simulink model "Absolute_Time_Temporal_Logic"  (R2018b)
settings: Solver=FixedStepDiscrete  StartTime=0.0  StopTime=40.0  FixedStep=1  RelTol=1e-3
undefined symbols (not defined in the file or in its folder): sigbuilder_block
settings Model: Creator=marwan  LastModifiedBy=marwan

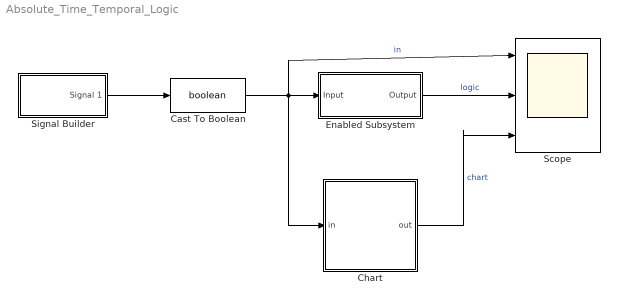
== system Absolute_Time_Temporal_Logic ==
  Cast To Boolean : DataTypeConversion  OutDataTypeStr=boolean
  Chart : Stateflow chart  TreatAsAtomicUnit=on
  Enabled Subsystem : Subsystem  TreatAsAtomicUnit=on
  Scope : Scope  NumInputPorts=3
  Signal Builder : Subsystem  Tag=STV Subsys  LoadFcn=sigbuilder_block('load');  StartFcn=sigbuilder_block('start');  StopFcn=sigbuilder_block('stop');  ClipboardFcn=sigbuilder_block('clipboard');  mask(Sigbuilder block){tuvar=[0:10]}
      mask help: Simulink:masks:SigbuilderBlock_MD
      mask init:
      | if ~strcmp(get_param(bdroot(gcbh),'SimulationStatus'),'stopped') tuvar = sigbuilder_block('maskInit'); end
      settings: CopyFcn=sigbuilder_block('copy');  DeleteFcn=sigbuilder_block('delete');  ModelCloseFcn=sigbuilder_block('modelClose');  PreSaveFcn=sigbuilder_block('preSave');  PauseFcn=sigbuilder_block('pause');  ContinueFcn=sigbuilder_block('continue');  NameChangeFcn=sigbuilder_block('namechange');  OpenFcn=sigbuilder_block('open',[369 79.5 565.5 358.5 ]);  CloseFcn=sigbuilder_block('close');
      mask Display: plot(0, 0, 100, 100,[2, 2, 32, 32, 2], [68, 8, 8, 68, 68],[32, 2], [38, 38], [32, 19, 2],[53, 60, 44], [32, 17, 17, 2],[16, 16, 31, 31]);txt = getActiveGroup(gcbh);text(2, 100, txt,'verticalAlignment', 'top');
  wires:
  Signal Builder/1(Signal 1) -> Cast To Boolean/1
  Cast To Boolean/1 -> Chart/1(in), Scope/1, Enabled Subsystem/1(Input)  "in"
  Enabled Subsystem/1(Output) -> Scope/2  "logic"
  Chart/1(out) -> Scope/3  "chart"

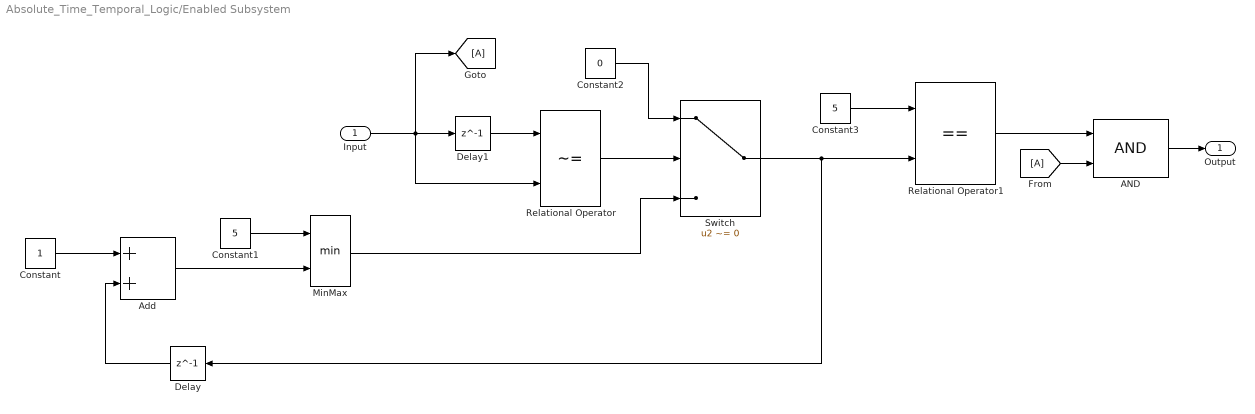
== system Absolute_Time_Temporal_Logic/Enabled Subsystem ==
  Input : Inport
  AND : Logic  IconShape=distinctive  AllPortsSameDT=off  OutDataTypeStr=boolean
  Add : Sum
  Constant : Constant
  Constant1 : Constant  Value=5
  Constant2 : Constant  Value=0
  Constant3 : Constant  Value=5
  Delay : Delay  DelayLength=1
  Delay1 : Delay  DelayLength=1
  MinMax : MinMax  Inputs=2
  Relational Operator : RelationalOperator  Operator=~=  OutDataTypeStr=boolean  RndMeth=Simplest
  Relational Operator1 : RelationalOperator  Operator===  OutDataTypeStr=boolean  RndMeth=Simplest
  Switch : Switch  Criteria=u2 ~= 0  Threshold=5
  Output : Outport
  wires:
  Delay/1 -> Add/2
  Constant/1 -> Add/1
  Constant1/1 -> MinMax/1
  Add/1 -> MinMax/2
  Input/1 -> [A], Relational Operator/2, Delay1/1
  Delay1/1 -> Relational Operator/1
  Relational Operator/1 -> Switch/2
  MinMax/1 -> Switch/3
  Constant2/1 -> Switch/1
  Constant3/1 -> Relational Operator1/1
  Switch/1 -> Delay/1, Relational Operator1/2
  Relational Operator1/1 -> AND/1
  [A] -> AND/2
  AND/1 -> Output/1

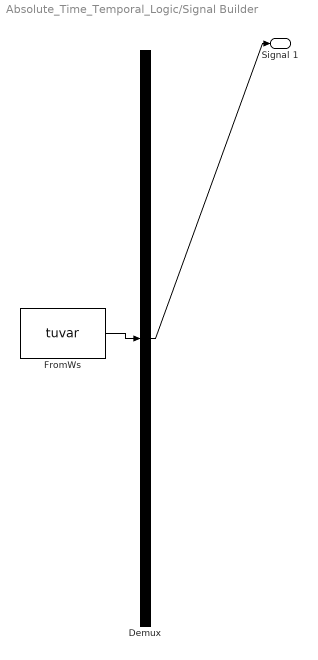
== system Absolute_Time_Temporal_Logic/Signal Builder ==
  Demux : Demux  Tag=STV Demux  Outputs=1
  FromWs : FromWorkspace  Tag=STV FromWs  VariableName=tuvar  SampleTime=0
      SigBuilderData=|
      | common.afterFinalStr = 'Extrapolate'
      | common.sampleTime = 0
      | dataSet.timeRange = [0 40]
      | dataSet.name = 'Group 1'
      | sbobj.Groups.Name = 'Group 1'
      | sbobj.Groups.Signals.Name = 'Signal 1'
      | sbobj.Groups.Signals.XData = [0 4.9 5 13 13.1 24.9 25 29 29.1 40]
      | sbobj.Groups.Signals.YData = [0 0 1 1 0 0 1 1 0 0]
      | sbobj.Groups.TimeRange = [0 40]
  Signal 1 : Outport  Tag=STV Outport
  wires:
  FromWs/1 -> Demux/1
  Demux/1 -> Signal 1/1

== stateflow chart Absolute_Time_Temporal_Logic/Chart ==
  state def
    en: out = false;
  state state2
    on after(5, sec):
    out = true;
  (default) -> def
  state2 -> def : [in == false]
  def -> state2 : [in == true]
  data: in input; out output
